simulink model "LQRFF"  (R2018a)
settings: Solver=VariableStepAuto  StartTime=0.0  StopTime=sim_time  RelTol=1e-3
values from neighbouring files (symbols this model uses):
  A = [0 V ... (first row only)    [kinematicLQR_FF.m]    (also in trailerKinematicsLQR.m = [0       0         0)
  B = [0 ... (first row only)    [kinematicLQR_FF.m]    (also in trailerKinematicsLQR.m = [vc./L2)
  C = eye(2)    [kinematicLQR_FF.m]    (also in trailerKinematicsLQR.m = eye(3))
  D = zeros(2, 1)    [kinematicLQR_FF.m]    (also in trailerKinematicsLQR.m = zeros(3, 1))
  F = M(1:n, end-l+1:end)    [kinematicLQR_FF.m]
  ICs = [y_IC deg2rad(0)]    [kinematicLQR_FF.m]    (also in trailerKinematicsLQR.m = [psi_1_IC; psi_2_IC; y_IC])
  L = 1.524    [kinematicLQR_FF.m]
  N = M(end-m+1:end, end-l+1:end)    [kinematicLQR_FF.m]
  V = 20    [kinematicLQR_FF.m]
  vehicleIC = [track_vector(1,1)-y_IC*sin(ICs(2)) track_vector(1,2)+y_IC*cos(ICs(2))]    [kinematicLQR_FF.m]
undefined symbols (not defined in the file or in its folder): K
settings Model: Creator=journeyman  LastModifiedBy=journeyman

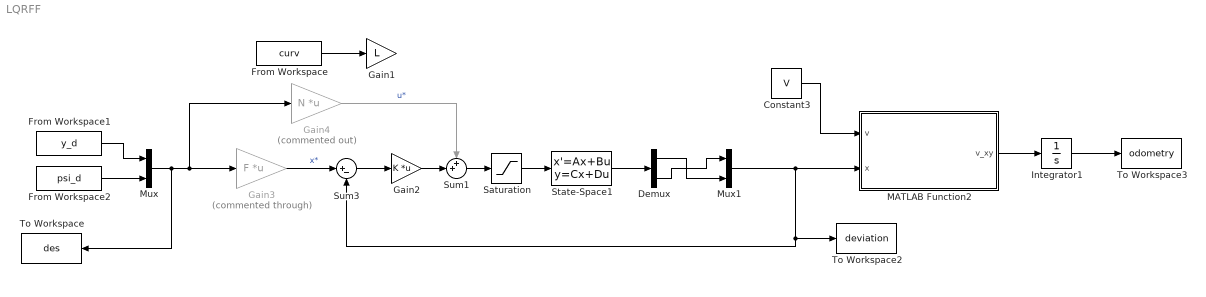
== system LQRFF ==
  Constant3 : Constant  Value=V
  Demux : Demux  Outputs=2
  From Workspace : FromWorkspace  VariableName=curv  SampleTime=0
  From Workspace1 : FromWorkspace  VariableName=y_d  SampleTime=0
  From Workspace2 : FromWorkspace  VariableName=psi_d  SampleTime=0
  Gain1 : Gain  Gain=L
  Gain2 : Gain  Gain=K  Multiplication=Matrix(K*u)
  Gain3 : Gain  Commented=through  Gain=F  Multiplication=Matrix(K*u)
  Gain4 : Gain  Commented=on  Gain=N  Multiplication=Matrix(K*u)
  Integrator1 : Integrator  InitialCondition=vehicleIC
  MATLAB Function2 : MATLAB Function  TreatAsAtomicUnit=on
  Mux : Mux  Inputs=2
  Mux1 : Mux  Inputs=2
  Saturation : Saturate  UpperLimit=deg2rad(30)  LowerLimit=deg2rad(-30)
  State-Space1 : StateSpace  A=A  B=B  C=C  D=D  InitialCondition=ICs
  Sum1 : Sum  Inputs=++|
  Sum3 : Sum  Inputs=|+-
  To Workspace : ToWorkspace  VariableName=des  SampleTime=-1
  To Workspace2 : ToWorkspace  VariableName=deviation  SampleTime=-1
  To Workspace3 : ToWorkspace  VariableName=odometry  SampleTime=-1
  wires:
  Integrator1/1 -> To Workspace3/1
  MATLAB Function2/1(v_xy) -> Integrator1/1
  Constant3/1 -> MATLAB Function2/1(v)
  From Workspace/1 -> Gain1/1
  Sum3/1 -> Gain2/1
  Gain3/1 -> Sum3/1  "x*"
  From Workspace1/1 -> Mux/1
  From Workspace2/1 -> Mux/2
  Sum1/1 -> Saturation/1
  Mux/1 -> To Workspace/1, Gain4/1, Gain3/1
  Gain2/1 -> Sum1/2
  Saturation/1 -> State-Space1/1
  Gain4/1 -> Sum1/1  "u*"
  State-Space1/1 -> Demux/1
  Demux/1 -> Mux1/2
  Demux/2 -> Mux1/1
  Mux1/1 -> To Workspace2/1, Sum3/2, MATLAB Function2/2(x)

== matlab function LQRFF/MATLAB Function2 ==
  data: v input; x input; v_xy output
function v_xy = DCM(v, x)

DCM = @(ang) [cos(ang) -sin(ang);
              sin(ang) cos(ang)];
          
v_xy = DCM(x(2))*[v; 0];
